simulink model "RobotTemplate"  (R2014b)
settings: configuration reference "SimulationConfig" (kept outside this file)
undefined symbols (not defined in the file or in its folder): gcbh, rmidispblock, tModel
libraries: NXTFcns x2, ControllersFcns x2
PreSaveFcn:
  | % Creates new data dictionary based on template.
  | 
  | projRoot = ETRoboconUtilities.getCheckoutRoot;
  | dictName = [bdroot 'Data.sldd'];
  | 
  | source = fullfile(projRoot,'templates','RobotTemplateData.sldd');
  | dest = fullfile(projRoot,'data_dictionaries',dictName);
  | 
  | if ~exist(dest) && ~isequal(bdroot,'RobotTemplate')
  |   copyfile(source,dest);
  |   disp(['Created new dictionary ' dictName ' in the data_dictionaries folder.']);
  |   set_param(bdroot,'DataDictionary', dictName);
  | end
Description:
  | ET Robocon 2014 robot template model.
  | 
  | Author:  Sebastian Castro
settings Model: DataDictionary=RobotTemplateData.sldd  ExtModeTrigDuration=2  Creator=mbiesiad  LastModifiedBy=scastro

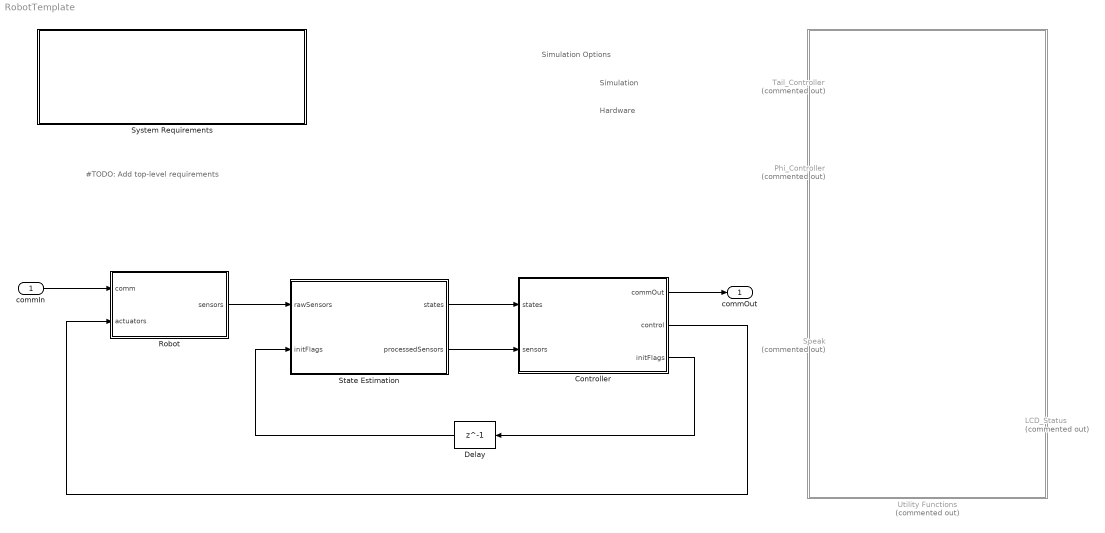
== system RobotTemplate ==
  note: #TODO:
      | Add top-level requirements
  note: Simulation Options
  note: Simulation
  note: Hardware
  commIn : Inport  OutDataTypeStr=Enum: Comm
  Controller : Stateflow chart  TreatAsAtomicUnit=on
  Delay : Delay  DelayLength=1  SampleTime=tModel
      settings: AttributesFormatString=Removes algebraic loop
  LCD_Status : NXTFcns/LCD_Status  Commented=on
  Phi_Controller : ControllersFcns/Phi_Controller  Commented=on
  Robot : Subsystem  Variant=on  VariantControl=Variant1  OverrideUsingVariant=SimulationVar
  Speak : NXTFcns/Speak  Commented=on
  State Estimation : Subsystem
  System Requirements : Subsystem  LoadFcn=rmidispblock('load',gcbh)  mask(System Requirements){id=SystemReq, title=System Requirements}
      mask prompts: title "Block Title"
      mask help: Lists the requirements for the current model.
      mask init:
      | id = 'SystemReq';
      | [w,h] = rmidispblock('display',gcbh);
      settings: CopyFcn=rmidispblock('create',gcbh)  DeleteFcn=rmidispblock('delete',gcbh)  ModelCloseFcn=rmidispblock('close',gcbh)  PreSaveFcn=rmidispblock('close',gcbh)  PostSaveFcn=rmidispblock('open',gcbh)  OpenFcn=rmidispblock('open',gcbh)  MoveFcn=rmidispblock('move',gcbh)
      mask Help: helpview(fullfile(docroot,'toolbox','slvnv','slvnv.map'),'systemrequirements')
      mask Display:
      | text(326/2,113-4,rmidispblock('title',gcbh),'horizontalAlignment','center','verticalAlignment','top')
      | text(w/2,h/2,'<No Requirements in System>','horizontalAlignment','center','verticalAlignment','top')
  Tail_Controller : ControllersFcns/Tail_Controller  Commented=on
  Utility Functions : Subsystem  Commented=on
  commOut : Outport  OutDataTypeStr=Enum: Comm
  wires:
  State Estimation/2(processedSensors) -> Controller/2(sensors)
  Robot/1(sensors) -> State Estimation/1(rawSensors)
  Controller/3(initFlags) -> Delay/1
  State Estimation/1(states) -> Controller/1(states)
  Delay/1 -> State Estimation/2(initFlags)
  Controller/2(control) -> Robot/2(actuators)
  Controller/1(commOut) -> commOut/1
  commIn/1 -> Robot/1(comm)

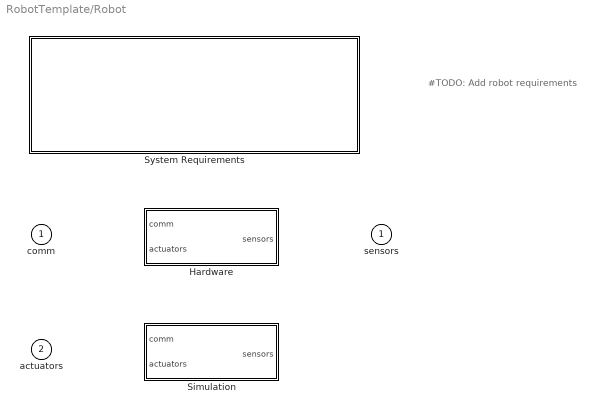
== system RobotTemplate/Robot ==
  note: #TODO:
      | Add robot requirements
  comm : Inport  OutDataTypeStr=Enum: Comm
  actuators : Inport  Port=2  OutDataTypeStr=Bus: ControlBus
  Hardware : Subsystem  VariantControl=HardwareVar
  Simulation : Subsystem  VariantControl=SimulationVar
  System Requirements : Subsystem  LoadFcn=rmidispblock('load',gcbh)  VariantControl=Variant  mask(System Requirements){id=SystemReq, title=System Requirements}
      mask prompts: title "Block Title"
      mask help: Lists the requirements for the current model.
      mask init:
      | id = 'SystemReq';
      | [w,h] = rmidispblock('display',gcbh);
      settings: CopyFcn=rmidispblock('create',gcbh)  DeleteFcn=rmidispblock('delete',gcbh)  ModelCloseFcn=rmidispblock('close',gcbh)  PreSaveFcn=rmidispblock('close',gcbh)  PostSaveFcn=rmidispblock('open',gcbh)  OpenFcn=rmidispblock('open',gcbh)  MoveFcn=rmidispblock('move',gcbh)
      mask Help: helpview(fullfile(docroot,'toolbox','slvnv','slvnv.map'),'systemrequirements')
      mask Display:
      | text(326/2,113-4,rmidispblock('title',gcbh),'horizontalAlignment','center','verticalAlignment','top')
      | text(w/2,h/2,'<No Requirements in System>','horizontalAlignment','center','verticalAlignment','top')
  sensors : Outport  OutDataTypeStr=Bus: SensorsBus

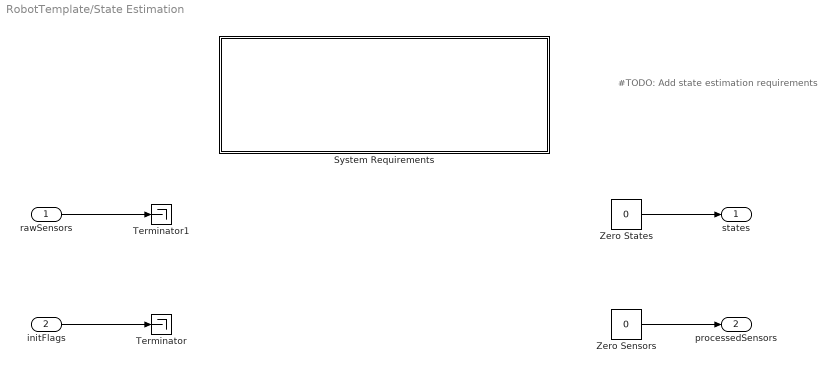
== system RobotTemplate/State Estimation ==
  note: #TODO:
      | Add state estimation requirements
  rawSensors : Inport  OutDataTypeStr=Bus: SensorsBus
  initFlags : Inport  Port=2  OutDataTypeStr=Bus: InitBus
  System Requirements : Subsystem  LoadFcn=rmidispblock('load',gcbh)  mask(System Requirements){id=SystemReq, title=System Requirements}
      mask prompts: title "Block Title"
      mask help: Lists the requirements for the current model.
      mask init:
      | id = 'SystemReq';
      | [w,h] = rmidispblock('display',gcbh);
      settings: CopyFcn=rmidispblock('create',gcbh)  DeleteFcn=rmidispblock('delete',gcbh)  ModelCloseFcn=rmidispblock('close',gcbh)  PreSaveFcn=rmidispblock('close',gcbh)  PostSaveFcn=rmidispblock('open',gcbh)  OpenFcn=rmidispblock('open',gcbh)  MoveFcn=rmidispblock('move',gcbh)
      mask Help: helpview(fullfile(docroot,'toolbox','slvnv','slvnv.map'),'systemrequirements')
      mask Display:
      | text(326/2,113-4,rmidispblock('title',gcbh),'horizontalAlignment','center','verticalAlignment','top')
      | text(w/2,h/2,'<No Requirements in System>','horizontalAlignment','center','verticalAlignment','top')
  Terminator : Terminator
  Terminator1 : Terminator
  Zero Sensors : Constant  Value=0  OutDataTypeStr=Bus: SensorsBus
  Zero States : Constant  Value=0  OutDataTypeStr=Bus: StatesBus
  states : Outport  OutDataTypeStr=Bus: StatesBus
  processedSensors : Outport  Port=2  OutDataTypeStr=Bus: SensorsBus
  wires:
  initFlags/1 -> Terminator/1
  rawSensors/1 -> Terminator1/1
  Zero Sensors/1 -> processedSensors/1
  Zero States/1 -> states/1

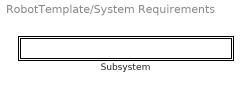
== system RobotTemplate/System Requirements ==
  Subsystem : Subsystem  mask{label=0, index=1}
      mask init:
      | label = rmidispblock('label',index);
      settings: OpenFcn=rmidispblock('openReq',gcbh);
      mask Display: text(0,0,label,'horizontalAlignment','left','verticalAlignment','bottom')

== system RobotTemplate/Utility Functions ==

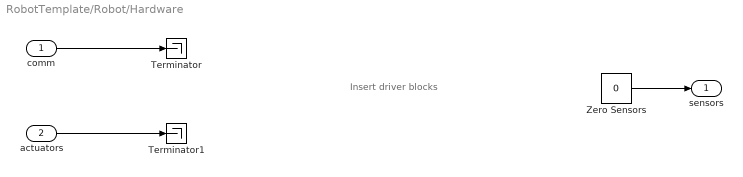
== system RobotTemplate/Robot/Hardware ==
  note: Insert driver blocks
  comm : Inport
  actuators : Inport  Port=2
  Terminator : Terminator
  Terminator1 : Terminator
  Zero Sensors : Constant  Value=0  OutDataTypeStr=Bus: SensorsBus
  sensors : Outport
  wires:
  Zero Sensors/1 -> sensors/1
  actuators/1 -> Terminator1/1
  comm/1 -> Terminator/1

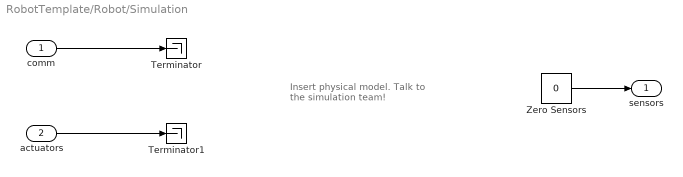
== system RobotTemplate/Robot/Simulation ==
  note: Insert physical model.
      | Talk to the simulation team!
  comm : Inport
  actuators : Inport  Port=2
  Terminator : Terminator
  Terminator1 : Terminator
  Zero Sensors : Constant  Value=0  OutDataTypeStr=Bus: SensorsBus
  sensors : Outport
  wires:
  Zero Sensors/1 -> sensors/1
  actuators/1 -> Terminator1/1
  comm/1 -> Terminator/1

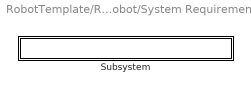
== system RobotTemplate/Robot/System Requirements ==
  Subsystem : Subsystem  mask{label=0, index=1}
      mask init:
      | label = rmidispblock('label',index);
      settings: OpenFcn=rmidispblock('openReq',gcbh);
      mask Display: text(0,0,label,'horizontalAlignment','left','verticalAlignment','bottom')

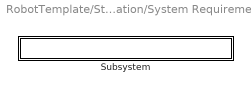
== system RobotTemplate/State Estimation/System Requirements ==
  Subsystem : Subsystem  mask{label=0, index=1}
      mask init:
      | label = rmidispblock('label',index);
      settings: OpenFcn=rmidispblock('openReq',gcbh);
      mask Display: text(0,0,label,'horizontalAlignment','left','verticalAlignment','bottom')

== system RobotTemplate/System Requirements/Subsystem ==

== system RobotTemplate/Robot/System Requirements/Subsystem ==

== system RobotTemplate/State Estimation/System Requirements/Subsystem ==

== stateflow chart RobotTemplate/Controller ==
  state initBuses [function]
    (default) -> (junction 186) : % Control bus
        | {
        | control.leftPWM = int8(0);
        | control.rightPWM = int8(0);
        | }
    (junction 186) -> (junction 187) : % Initialization flags
        | {
        | initFlags.encoder = false;
        | initFlags.gyro = false;
        | }
  state DefaultState
    % Add control logic here.
  note: #TODO
      | Add requirements to Stateflow objects
      | by right-clicking and selecting the
      | Requirements Traceability option.
  (default) -> DefaultState : % Initialize data
      | {
      | initBuses();
      | commOut = Comm.NONE;
      | }
  data: commOut output Enum: Comm size=1; control output Bus: ControlBus size=1; states input Bus: StatesBus size=1; sensors input Bus: SensorsBus size=1; initFlags output Bus: InitBus size=1
